simulink model "sensor_fusion_r2024_version"  (R2024b)
settings: Solver=VariableStepAuto  StartTime=0.0  StopTime=10.0  RelTol=1e-3
settings Model: Creator=v shruthi  LastModifiedBy=v shruthi
settings ConfigComp: CovBoundaryAbsTol=1.0e-5

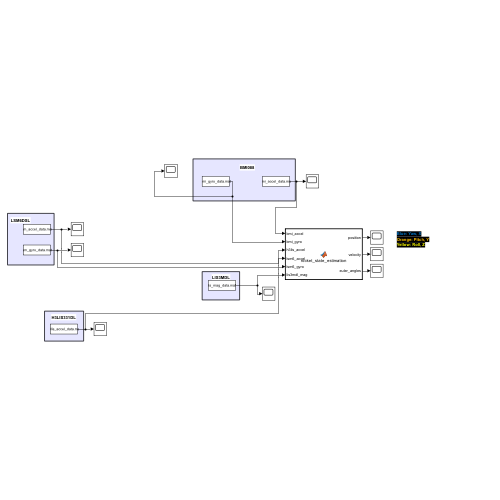
[thumbnail: Simulink's stored preview of the top-level diagram]
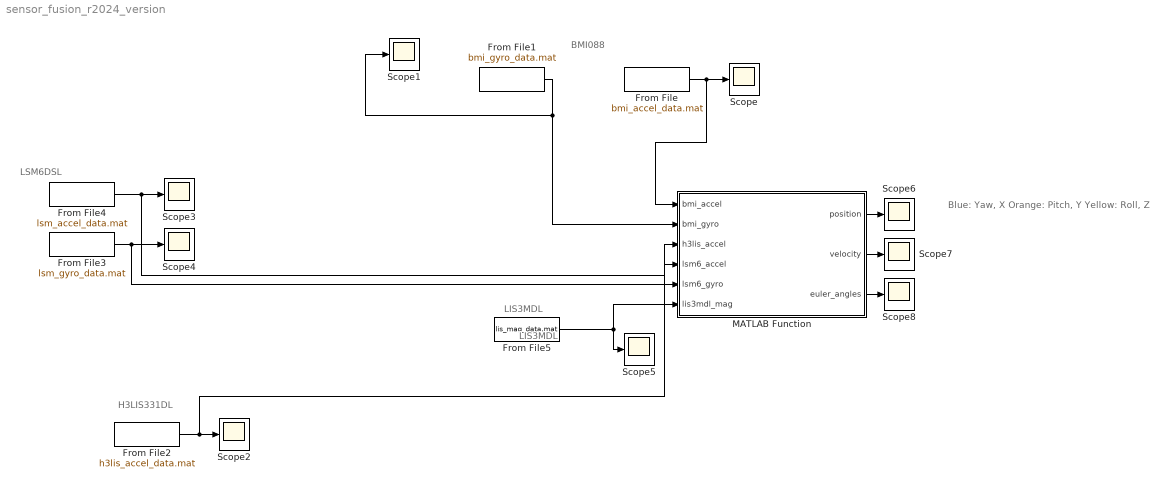
== system sensor_fusion_r2024_version ==
  note: BMI088
  note: LSM6DSL
  note: Blue: Yaw, X
      | Orange: Pitch, Y
      | Yellow: Roll, Z
  note: LIS3MDL
  note: LIS3MDL
  note: H3LIS331DL
  From File : FromFile  FileName=bmi_accel_data.mat  SampleTime=0
  From File1 : FromFile  FileName=bmi_gyro_data.mat  SampleTime=0
  From File2 : FromFile  FileName=h3lis_accel_data.mat  SampleTime=0
  From File3 : FromFile  FileName=lsm_gyro_data.mat  SampleTime=0
  From File4 : FromFile  FileName=lsm_accel_data.mat  SampleTime=0
  From File5 : FromFile  FileName=lis_mag_data.mat  SampleTime=0
  MATLAB Function : MATLAB Function  TreatAsAtomicUnit=on
  Scope{,1..8} (9 alike) : Scope
  wires:
  From File/1 -> MATLAB Function/1(bmi_accel), Scope/1
  From File1/1 -> MATLAB Function/2(bmi_gyro), Scope1/1
  From File2/1 -> MATLAB Function/3(h3lis_accel), Scope2/1
  From File3/1 -> MATLAB Function/5(lsm6_gyro), Scope4/1
  From File4/1 -> MATLAB Function/4(lsm6_accel), Scope3/1
  From File5/1 -> Scope5/1, MATLAB Function/6(lis3mdl_mag)
  MATLAB Function/1(position) -> Scope6/1
  MATLAB Function/2(velocity) -> Scope7/1
  MATLAB Function/3(euler_angles) -> Scope8/1

== matlab function sensor_fusion_r2024_version/MATLAB Function ==
  data: bmi_accel input; position output; bmi_gyro input; h3lis_accel input; lsm6_accel input; lsm6_gyro input; lis3mdl_mag input; velocity output; euler_angles output
function [position, velocity, euler_angles] = rocket_state_estimation(...
    bmi_accel, bmi_gyro, h3lis_accel, lsm6_accel, lsm6_gyro, lis3mdl_mag)
    
    %#codegen % Required for Simulink code generation
    
    % Initialize persistent variables with explicit sizes
    persistent x dt q_orientation mag_filtered
    if isempty(x)
        % State vector: [position (3); velocity (3)]
        x = zeros(6,1); % 6x1 column vector
        dt = 0.0025;    % 400Hz sample rate (0.0025s)
        q_orientation = [1; 0; 0; 0]; % 4x1 quaternion (w,x,y,z)
        mag_filtered = [1; 0; 0];     % 3x1 magnetometer vector
    end
    
    % SAFE INPUT HANDLING - guarantees 3-element vectors
    % BMI Accelerometer
    bmi_accel_1 = bmi_accel(1);
    bmi_accel_2 = if_has_element(bmi_accel, 2);
    bmi_accel_3 = if_has_element(bmi_accel, 3);
    
    % LSM6 Accelerometer
    lsm6_accel_1 = lsm6_accel(1);
    lsm6_accel_2 = if_has_element(lsm6_accel, 2);
    lsm6_accel_3 = if_has_element(lsm6_accel, 3);
    
    % Average accelerometers
    accel_1 = 0.5*(bmi_accel_1 + lsm6_accel_1);
    accel_2 = 0.5*(bmi_accel_2 + lsm6_accel_2);
    accel_3 = 0.5*(bmi_accel_3 + lsm6_accel_3);
    
    % High-G accelerometer
    h3lis_1 = h3lis_accel(1);
    h3lis_2 = if_has_element(h3lis_accel, 2);
    h3lis_3 = if_has_element(h3lis_accel, 3);
    
    % Thrust detection (switch to high-G accelerometer)
    if sqrt(h3lis_1^2 + h3lis_2^2 + h3lis_3^2) > 2*9.81
        accel_1 = h3lis_1;
        accel_2 = h3lis_2;
        accel_3 = h3lis_3;
    end
    
    % Gyro inputs with safe access
    gyro_1 = 0.5*(bmi_gyro(1) + lsm6_gyro(1));
    gyro_2 = 0.5*(if_has_element(bmi_gyro, 2) + if_has_element(lsm6_gyro, 2));
    gyro_3 = 0.5*(if_has_element(bmi_gyro, 3) + if_has_element(lsm6_gyro, 3));
    
    % Magnetometer with safe access
    mag_1 = lis3mdl_mag(1);
    mag_2 = if_has_element(lis3mdl_mag, 2);
    mag_3 = if_has_element(lis3mdl_mag, 3);
    
    % QUATERNION ROTATION (manual implementation)
    qw = q_orientation(1);
    qx = q_orientation(2);
    qy = q_orientation(3);
    qz = q_orientation(4);
    
    % Rotation matrix elements
    R11 = 1 - 2*(qy^2 + qz^2);
    R12 = 2*(qx*qy - qw*qz);
    R13 = 2*(qx*qz + qw*qy);
    
    R21 = 2*(qx*qy + qw*qz);
    R22 = 1 - 2*(qx^2 + qz^2);
    R23 = 2*(qy*qz - qw*qx);
    
    R31 = 2*(qx*qz - qw*qy);
    R32 = 2*(qy*qz + qw*qx);
    R33 = 1 - 2*(qx^2 + qy^2);
    
    % Gravity in body frame
    gravity_1 = R13*9.81;
    gravity_2 = R23*9.81;
    gravity_3 = R33*9.81;
    
    % Linear acceleration
    linear_accel_1 = accel_1 - gravity_1;
    linear_accel_2 = accel_2 - gravity_2;
    linear_accel_3 = accel_3 - gravity_3;
    
    % STATE PROPAGATION
    % Position update
    x(1) = x(1) + x(4)*dt;
    x(2) = x(2) + x(5)*dt;
    x(3) = x(3) + x(6)*dt;
    
    % Velocity update
    x(4) = x(4) + linear_accel_1*dt;
    x(5) = x(5) + linear_accel_2*dt;
    x(6) = x(6) + linear_accel_3*dt;
    
    % QUATERNION INTEGRATION
    q_dot_w = 0.5 * (-qx*gyro_1 - qy*gyro_2 - qz*gyro_3);
    q_dot_x = 0.5 * (qw*gyro_1 - qz*gyro_2 + qy*gyro_3);
    q_dot_y = 0.5 * (qz*gyro_1 + qw*gyro_2 - qx*gyro_3);
    q_dot_z = 0.5 * (-qy*gyro_1 + qx*gyro_2 + qw*gyro_3);
    
    q_orientation(1) = q_orientation(1) + q_dot_w*dt;
    q_orientation(2) = q_orientation(2) + q_dot_x*dt;
    q_orientation(3) = q_orientation(3) + q_dot_y*dt;
    q_orientation(4) = q_orientation(4) + q_dot_z*dt;
    
    % Normalization
    norm_q = sqrt(q_orientation(1)^2 + q_orientation(2)^2 + ...
                 q_orientation(3)^2 + q_orientation(4)^2);
    q_orientation = q_orientation/max(norm_q, eps); % Avoid division by zero
    
    % MAGNETOMETER PROCESSING
    mag_filtered(1) = 0.9*mag_filtered(1) + 0.1*mag_1;
    mag_filtered(2) = 0.9*mag_filtered(2) + 0.1*mag_2;
    mag_filtered(3) = 0.9*mag_filtered(3) + 0.1*mag_3;
    
    mag_norm = sqrt(mag_filtered(1)^2 + mag_filtered(2)^2 + mag_filtered(3)^2);
    if mag_norm > eps
        mag_norm_x = mag_filtered(1)/mag_norm;
        mag_norm_y = mag_filtered(2)/mag_norm;
    else
        mag_norm_x = 1;
        mag_norm_y = 0;
    end
    
    % EULER ANGLES CONVERSION
    q0 = q_orientation(1);
    q1 = q_orientation(2);
    q2 = q_orientation(3);
    q3 = q_orientation(4);
    
    % 1. Clamp the asin() argument to valid range [-1, 1]
    sin_pitch = 2*(q0*q2 - q3*q1);
    sin_pitch = min(max(sin_pitch, -1), 1); % Force within [-1, 1]
    
    % 2. Calculate pitch with protection
    if abs(sin_pitch) >= 1
        pitch = sign(sin_pitch) * pi/2; % ±90° if at limits
    else
        pitch = asin(sin_pitch);
    end
    
    % 3. Special handling at gimbal lock (pitch near ±90°)
    if abs(pitch) > 0.9999*pi/2
        yaw = atan2(2*(q1*q2 - q0*q3), q0^2 - q1^2 + q2^2 - q3^2);
        roll = 0; % Roll undefined at gimbal lock
    else
        yaw = atan2(mag_norm_y, mag_norm_x);
        roll = atan2(2*(q0*q1 + q2*q3), 1 - 2*(q1^2 + q2^2));
    end
        
    % OUTPUTS
    position = [x(1); x(2); x(3)];     % [North; East; Down] (m)
    velocity = [x(4); x(5); x(6)];     % [Vn; Ve; Vd] (m/s)
    euler_angles = [yaw; pitch; roll]; % [Yaw; Pitch; Roll] (rad)
end

% Helper function for safe array access
function val = if_has_element(arr, idx)
    if length(arr) >= idx
        val = arr(idx);
    else
        val = 0; % Default value if element doesn't exist
    end
end
